simulink model "ESTHeatingSystem"  (R2017a)
settings: Solver=FixedStepAuto  StartTime=0.0  StopTime=100  FixedStep=0.1  MaxStep=0.1  RelTol=1e-3
PreLoadFcn:
  | load ('parameters\parameters.mat');
libraries: simulink x1
settings Model: Creator=xiaodong  LastModifiedBy=xiaodong
settings DataIOCC: SaveFormat=Array  SaveTime=off

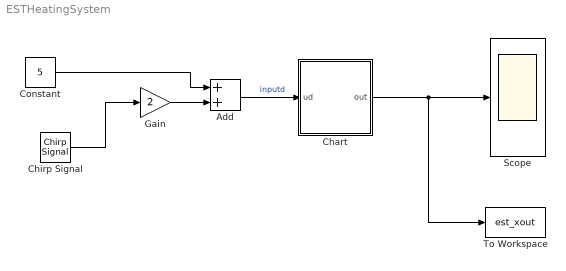
== system ESTHeatingSystem ==
  Add : Sum
  Chart : Stateflow chart  TreatAsAtomicUnit=on
  Chirp Signal : simulink/Sources/Chirp Signal  f1=0.001  T=100  f2=0.01
  Constant : Constant  Value=5
  Gain : Gain  Gain=2
  Scope : Scope
  To Workspace : ToWorkspace  VariableName=est_xout  SampleTime=-1
  wires:
  Gain/1 -> Add/2
  Constant/1 -> Add/1
  Chirp Signal/1 -> Gain/1
  Add/1 -> Chart/1(ud)  "inputd"
  Chart/1(out) -> Scope/1, To Workspace/1

== stateflow chart ESTHeatingSystem/Chart ==
  state M2
    entry:
    A2 =[0.9901, 0.0030, 0.0039;
    0.0021, 0.9897, 0.0052;
    0.0041, 0.0050, 0.9860];
    Bd2 = [0.0030; 0.0020; 0.0050];
    Bc2=[0.0000;  0.0836; 0.0000];
    during:
    x= FnM(A2, x)+FnM(Bd2,ud)+Bc2;
    out = x;
  state M5
    entry:
    A3 = [0.9947 	-0.0077    0.0093;
    0.0030	0.9901	    0.0050;
    0.0039	0.0049	    0.9861];
    Bd3 = [0.0023; 0.0020; 0.0050];
    Bc3 = [0.0914; 0.0000; 0.0000];
    during:
    x = FnM(A3,x)+Bd3*ud+Bc3;
    out = x;
  state M4
    entry:
    A1 = [0.9901    0.0030    0.0040;
    0.0030    0.9901    0.0049;
    0.0039    0.0049    0.9861];
    Bd1 = [0.0030; 0.0020; 0.0050];
    Bc1 = [0.0000; 0.0000; 0.1098];
    during:
    x =FnM(A1,x)+Bd1*ud+Bc1;
    out = x;
  state M236
    entry:
    A4 = [0.9900    0.0030    0.0093;
    0.0030    0.9901    0.0049;
    0.0039    0.0049    0.9861];
    Bd4 = [0.0030; 0.0020; 0.0050];
    Bc4 = [0.0011; 0.0000; 0.0018];
    during:
    x= FnM(A4,x)+Bd4*ud+Bc4;
    out = x;
  state M262
    entry:
    A4 = [0.9900    0.0030    0.0093;
    0.0030    0.9901    0.0049;
    0.0039    0.0049    0.9861];
    Bd4 = [0.0030; 0.0020; 0.0050];
    Bc4 = [0.0011; 0.0000; 0.0018];
    during:
    x = FnM(A4,x)+Bd4*ud+Bc4;
    out = x;
  state M267
    entry:
    A4 = [0.9900    0.0030    0.0093;
    0.0030    0.9901    0.0049;
    0.0039    0.0049    0.9861];
    Bd4 = [0.0030; 0.0020; 0.0050];
    Bc4 = [0.0011; 0.0000; 0.0018];
    during:
    x = FnM(A4,x)+Bd4*ud+Bc4;
    out = x;
  M5 -> M2 [order 2] : [(-0.3309*x(1)+0.3292*x(2)+ 0.0016*x(3)+ 1<=0) && (-0.0641*x(2)+1>=0)]
  (default) -> M2 : {x=[15;15;15]; out=x;}
  M2 -> M4 [order 1] : [(-0.4794*x(2)+0.4770*x(3) + 1<=0) &&(0.0014*x(1)-0.0659*x(3)+ 1>=0)]
  M4 -> M5 [order 2] : [(0.4884*x(1)+ 0.0013*x(2)-0.4901*x(3)+ 1<=0) && (-0.0627*x(1)+ 1>=0)]
  M236 -> M2 : [-0.0527*x(2)+ 1>=0]
  M2 -> M236 [order 2] : [-0.0480*x(2)+ 1<=0]
  M267 -> M5 : [-0.0496*x(1)+ 1>=0]
  M5 -> M267 [order 1] : [-0.0475*x(1)+ 1<=0]
  M262 -> M4 : [-0.0539*x(3)+ 1>=0]
  M4 -> M262 [order 1] : [-0.0456*x(3)+ 1<=0]
  data: u1 function_input; u2 function_input; y function_output; A2 local double size=[3,3]; Bd2 local size=[3,1]; Bc2 local size=[3,1]; x local size=3 =[10;10;10]; A3 local size=[3,3]; Bd3 local size=[3,1]; Bc3 local size=[3,1]; ud input size=1; Bd4 local size=[3,1]; Bd1 local size=[3,1]; Bc4 local size=[3,1]; Bc1 local size=[3,1]; A4 local size=[3,3]; A1 local size=[3,3]; out output size=3 =[15 15 15]'
  function y = FnM(u1, u2):
    | function y = FnM(u1, u2)
    | y = u1*u2;
